simulink model "Fpump"  (R2025b)
settings: Solver=ode1be  StartTime=0.0  StopTime=300  FixedStep=0.03  RelTol=1e-3
undefined symbols (not defined in the file or in its folder): DiscIntNeverNeededParam
settings Model: Creator=peace  LastModifiedBy=peace
settings RTWCC: GPUComputeCapability=3.5

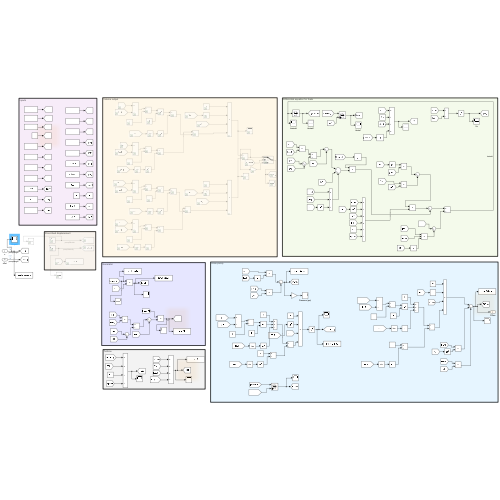
[thumbnail: Simulink's stored preview of the top-level diagram]
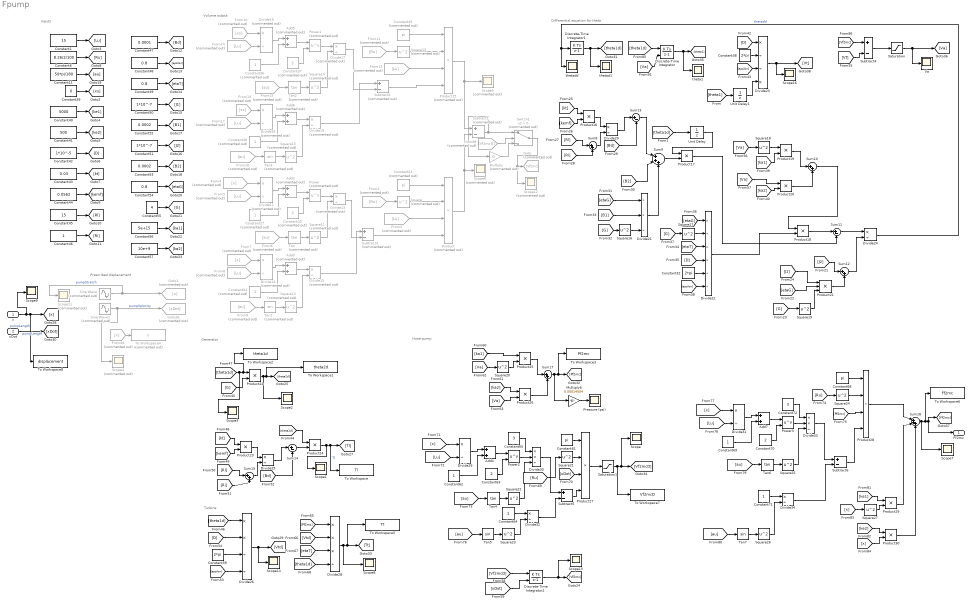
== system Fpump ==
  note: Turbine
  note: Hose-pump
  note: Generator
  note: Differential equation for theta
  note: Volume output
  note: Prescribed displacement
  note: Inputs
  x : Inport
  xDot : Inport  Port=2
  Add{2..3,5..6} (4 alike) : Sum  Commented=on
  Add4 : Sum
  Add7 : Sum
  Constant1 : Constant  Value=15
  Constant11 : Constant  Value=50*pi/180
  Constant23 : Constant  Commented=on  Value=pi
  Constant{27,34,36,38} (4 alike) : Constant  Commented=on
  Constant32 : Constant  Value=2*pi
  Constant33 : Constant  Commented=on  Value=3
  Constant35 : Constant  Commented=on  Value=pi
  Constant37 : Constant  Commented=on  Value=3
  Constant39 : Constant  Value=0
  Constant40 : Constant  Value=5000
  Constant41 : Constant  Value=500
  Constant42 : Constant  Value=1*10^-5
  Constant43 : Constant  Value=0.03
  Constant44 : Constant  Value=0.0562
  Constant45 : Constant  Value=15
  Constant{46,62,64,69,71} (5 alike) : Constant
  Constant47 : Constant  Value=0.0001
  Constant48 : Constant  Value=0.8
  Constant49 : Constant  Value=0.8
  Constant50 : Constant  Value=1*10^-7
  Constant51 : Constant  Value=1*10^-7
  Constant52 : Constant  Value=0.0002
  Constant53 : Constant  Value=0.0002
  Constant54 : Constant  Value=0.8
  Constant55 : Constant  Value=4
  Constant56 : Constant  Value=5e+15
  Constant57 : Constant  Value=10e+9
  Constant58 : Constant  Value=2*pi
  Constant59 : Constant  Value=2*pi
  Constant6 : Constant  Value=8.26/2/100
  Constant61 : Constant  Value=pi
  Constant63 : Constant  Value=2
  Constant65 : Constant  Value=3
  Constant68 : Constant  Value=pi
  Constant70 : Constant  Value=2
  Constant72 : Constant  Value=3
  Discrete-Time Integrator : DiscreteIntegrator  ExternalReset=falling  SampleTime=-1  ICPrevOutput=DiscIntNeverNeededParam  ICPrevScaledInput=DiscIntNeverNeededParam
  Discrete-Time Integrator1 : DiscreteIntegrator  SampleTime=-1  ICPrevOutput=DiscIntNeverNeededParam  ICPrevScaledInput=DiscIntNeverNeededParam
  Discrete-Time Integrator2 : DiscreteIntegrator  ExternalReset=falling  SampleTime=-1  ICPrevOutput=DiscIntNeverNeededParam  ICPrevScaledInput=DiscIntNeverNeededParam
  Divide{11,13..19} (8 alike) : Product  Commented=on  Inputs=*/
  Divide{20,24..25,29,31..32,34} (7 alike) : Product  Inputs=*/
  Divide21 : Product  Inputs=**/
  Divide22 : Product  Inputs=*/**//
  Divide23 : Product  Inputs=*//*
  Divide26 : Product  Inputs=**//
  Divide28 : Product  Inputs=***/
  Divide30 : Product  Inputs=**/
  Divide33 : Product  Inputs=**/
  From10 : From  Commented=on  GotoTag=xs
  From11 : From  Commented=on  GotoTag=Ru
  From{3,5,8,12,14,17} (6 alike) : From  Commented=on  GotoTag=Lu
  From13 : From  Commented=on  GotoTag=xs
  From{6,9,15,18} (4 alike) : From  Commented=on  GotoTag=au
  From2 : From  Commented=on  GotoTag=Ru
  From4 : From  Commented=on  GotoTag=x
  From64 : From  Commented=on  GotoTag=x
  From7 : From  Commented=on  GotoTag=x
  From89 : From  Commented=on  GotoTag=Vf2mcD
  Goto : Goto  Commented=on  GotoTag=Vf2mc
  Goto1 : Goto  Commented=on  GotoTag=x
  Goto26 : Goto  Commented=on  GotoTag=xDot
  Multiply : Gain  Commented=on  Gain=0
  Multiply6 : Gain  Gain=0.00014504
  Power : Math  Commented=on  Operator=pow
  Power1 : Math  Commented=on  Operator=pow
  Power2 : Math  Operator=pow
  Power3 : Math  Operator=pow
  Pressure (psi) : Scope
      settings: ActiveDisplayYMinimum=-78.359380613030112  ActiveDisplayYMaximum=705.23442551727112  DataLoggingVariableName=ScopeData10
  Product : Product  Commented=on  Inputs=4
  Product15 : Product  Commented=on  Inputs=4
  Product{16..20,22..26,29..30} (12 alike) : Product
  Product21 : Product  Inputs=3
  Product27 : Product  Inputs=4
  Product28 : Product  Inputs=4
  Saturation : Saturate  UpperLimit=Inf  LowerLimit=0
  Saturation1 : Saturate  UpperLimit=Inf  LowerLimit=0
  Scope{,1..3,7..9,13..14,16} (10 alike) : Scope
      Scope settings: ActiveDisplayYMinimum=-0.0003969816965604729  ActiveDisplayYMaximum=0.0035728352690442573  DataLoggingVariableName=ScopeData9
      Scope1 settings: ActiveDisplayYMinimum=-1  ActiveDisplayYMaximum=1
      Scope13 settings: ActiveDisplayYMinimum=-1  ActiveDisplayYMaximum=1  DataLoggingVariableName=ScopeData15
      Scope14 settings: ActiveDisplayYMinimum=-4.3E-5  ActiveDisplayYMaximum=4E-5  DataLoggingVariableName=ScopeData4
      Scope16 settings: ActiveDisplayYMinimum=-1  ActiveDisplayYMaximum=1  DataLoggingVariableName=ScopeData16
      Scope2 settings: ActiveDisplayYMinimum=-807.31564  ActiveDisplayYMaximum=7200.0744  DataLoggingVariableName=ScopeData2
      Scope3 settings: ActiveDisplayYMinimum=-201.82891  ActiveDisplayYMaximum=1800.0186  DataLoggingVariableName=ScopeData3
      Scope7 settings: ActiveDisplayYMinimum=-3.4318250735998834E+23  ActiveDisplayYMaximum=1.6249217794143435E+24  DataLoggingVariableName=ScopeData13
      Scope8 settings: ActiveDisplayYMinimum=-0.85985  ActiveDisplayYMaximum=7.73866  DataLoggingVariableName=ScopeData11
      Scope9 settings: DataLoggingVariableName=ScopeData7
  Scope{4..6,11..12} (5 alike) : Scope  Commented=on
      Scope11 settings: ActiveDisplayYMinimum=-0.24999999999999994  ActiveDisplayYMaximum=2.25  DataLoggingVariableName=ScopeData6
      Scope12 settings: ActiveDisplayYMinimum=-0.00094087179819930442  ActiveDisplayYMaximum=0.0084678461837937417  DataLoggingVariableName=ScopeData2
      Scope4 settings: ActiveDisplayYMinimum=-1  ActiveDisplayYMaximum=1
      Scope5 settings: ActiveDisplayYMinimum=0.07038  ActiveDisplayYMaximum=0.09038  DataLoggingVariableName=ScopeData5
      Scope6 settings: ActiveDisplayYMinimum=0.07191  ActiveDisplayYMaximum=0.08132  DataLoggingVariableName=ScopeData6
  Sine Wave : Sin  Commented=on  Bias=1  Frequency=2*pi/8  Phase=3*pi/2  SampleTime=0
  Sine Wave1 : Sin  Commented=on  Amplitude=1*2*pi/8  Frequency=2*pi/8  SampleTime=0
  Square{,11..15} (6 alike) : Math  Commented=on  Operator=square
  Square{16..27} (12 alike) : Math  Operator=square
  Subtract1 : Sum  Commented=on  Inputs=+-
  Subtract2 : Sum  Commented=on  Inputs=+-
  Subtract3 : Sum  Commented=on  Inputs=+-
  Subtract4 : Sum  Inputs=+-
  Subtract5 : Sum  Inputs=+-
  Subtract6 : Sum  Inputs=+-
  Sum{8,10,12,15,17} (5 alike) : Sum  Inputs=|++
  Sum11 : Sum  Inputs=|+-
  Sum13 : Sum  Inputs=|+-
  Sum14 : Sum  Inputs=|+-
  Sum18 : Sum  Inputs=|+++
  Sum9 : Sum  Inputs=|+++
  Switch1 : Switch  Commented=on  Criteria=u2 > Threshold  SaturateOnIntegerOverflow=off  InputSameDT=off
  Tan : Trigonometry  Commented=on  Operator=tan
  Tan1 : Trigonometry  Commented=on
  Tan2 : Trigonometry  Commented=on  Operator=tan
  Tan3 : Trigonometry  Commented=on
  Tan4 : Trigonometry  Operator=tan
  Tan5 : Trigonometry
  Tan6 : Trigonometry  Operator=tan
  Tan7 : Trigonometry
  To Workspace : ToWorkspace  VariableName=Tl  SampleTime=-1
  To Workspace1 : ToWorkspace  VariableName=theta2d  SampleTime=-1
  To Workspace2 : ToWorkspace  VariableName=theta1d  SampleTime=-1
  To Workspace3 : ToWorkspace  VariableName=Pf2mc  SampleTime=-1
  To Workspace4 : ToWorkspace  Commented=on  VariableName=x  SaveFormat=Structure With Time  SampleTime=-1
  To Workspace5 : ToWorkspace  VariableName=Tt  SampleTime=-1
  To Workspace6 : ToWorkspace  VariableName=Ff2mc  SampleTime=-1
  To Workspace7 : ToWorkspace  VariableName=Vf2mcD  SampleTime=-1
  To Workspace8 : ToWorkspace  VariableName=displacement  SampleTime=-1
  Unit Delay : UnitDelay  SampleTime=-1  HasFrameUpgradeWarning=on
  Unit Delay1 : UnitDelay  SampleTime=-1  HasFrameUpgradeWarning=on
  Va : Scope
      settings: ActiveDisplayYMinimum=-4E-6  ActiveDisplayYMaximum=3.2E-5  DataLoggingVariableName=ScopeData3
  theta1 : Scope
      settings: ActiveDisplayYMinimum=-472.7300411952894  ActiveDisplayYMaximum=4254.5703707576058  DataLoggingVariableName=ScopeData14
  thetad1 : Scope
      settings: ActiveDisplayYMinimum=-90.070687849635348  ActiveDisplayYMaximum=697.42712539466106  DataLoggingVariableName=ScopeData12
  thetadd : Scope
      settings: ActiveDisplayYMinimum=-1  ActiveDisplayYMaximum=1
  Ff2mc : Outport
  wires:
  Sine Wave/1 -> Scope11/1, Goto1/1  "pumpStretch"
  Constant11/1 -> [au]
  Constant1/1 -> [Lu]
  Constant6/1 -> [Ru]
  From2/1 -> Square/1
  Constant23/1 -> Product/1
  Square/1 -> Product/2
  From3/1 -> Product/3
  From5/1 -> Divide11/2
  Divide11/1 -> Add2/1
  Constant27/1 -> Add2/2
  Add2/1 -> Power/1
  Constant33/1 -> Power/2
  Power/1 -> Divide13/1
  From6/1 -> Tan/1
  Tan/1 -> Square11/1
  Square11/1 -> Divide13/2
  Tan1/1 -> Square12/1
  From9/1 -> Tan1/1
  Constant34/1 -> Add3/2
  Square12/1 -> Divide15/2
  From8/1 -> Divide14/2
  From7/1 -> Divide14/1
  Add3/1 -> Divide15/1
  Divide14/1 -> Add3/1
  Divide13/1 -> Subtract3/2
  Divide15/1 -> Subtract3/1
  Subtract3/1 -> Product/4
  Tan2/1 -> Square14/1
  Subtract2/1 -> Product15/4
  From15/1 -> Tan2/1
  From10/1 -> Divide16/1
  Divide19/1 -> Subtract2/1
  From14/1 -> Divide16/2
  Divide18/1 -> Add6/1
  From13/1 -> Divide18/1
  From17/1 -> Divide18/2
  Tan3/1 -> Square15/1
  Constant38/1 -> Add6/2
  From18/1 -> Tan3/1
  Constant37/1 -> Power1/2
  Square13/1 -> Product15/2
  Constant36/1 -> Add5/2
  Constant35/1 -> Product15/1
  From11/1 -> Square13/1
  Square14/1 -> Divide17/2
  Power1/1 -> Divide17/1
  Add5/1 -> Power1/1
  Add6/1 -> Divide19/1
  Square15/1 -> Divide19/2
  From12/1 -> Product15/3
  Divide16/1 -> Add5/1
  Product15/1 -> Subtract1/1, Scope5/1
  Constant39/1 -> [xs]
  From4/1 -> Divide11/1
  Divide17/1 -> Subtract2/2
  Product/1 -> Subtract1/2, Scope6/1
  Constant40/1 -> [ke1]
  Constant41/1 -> [ke2]
  Constant42/1 -> [D]
  Constant43/1 -> [kt]
  Constant44/1 -> [kemf]
  Constant46/1 -> [Ri]
  Constant47/1 -> [Bd]
  Constant45/1 -> [Rl]
  Constant48/1 -> [epsilon]
  Constant49/1 -> [etaT]
  Constant50/1 -> [J1]
  Constant52/1 -> [B1]
  Constant51/1 -> [J2]
  Constant53/1 -> [B2]
  Constant54/1 -> [etaG]
  Constant55/1 -> [G]
  [Rl] -> Sum8/1
  [Ri] -> Sum8/2
  [kt] -> Product16/1
  [kemf] -> Product16/2
  Product16/1 -> Divide20/1
  Sum8/1 -> Divide20/2
  Divide20/1 -> Sum13/1
  [Bd] -> Sum13/2
  [B2] -> Sum9/2
  [etaG] -> Divide21/1
  [G] -> Square16/1
  Square16/1 -> Divide21/3
  [B1] -> Divide21/2
  Sum9/1 -> Product17/2
  Square17/1 -> Divide22/2
  [G] -> Square17/1
  [etaG] -> Divide22/1
  [etaT] -> Divide22/3
  [D] -> Divide22/4
  Constant32/1 -> Divide22/5
  [epsilon] -> Divide22/6
  Constant56/1 -> [ka1]
  Constant57/1 -> [ka2]
  Divide22/1 -> Product18/2
  [D] -> Divide23/1
  [epsilon] -> Divide23/3
  Constant58/1 -> Divide23/2
  Square18/1 -> Product19/1
  [ka1] -> Product19/2
  [ka2] -> Product20/2
  Product19/1 -> Sum10/1
  Product20/1 -> Sum10/2
  Sum10/1 -> Product18/1
  Product18/1 -> Sum11/1
  Product17/1 -> Sum11/2
  Sum11/1 -> Divide24/1
  [J1] -> Product21/1
  [G] -> Square19/1
  [etaG] -> Product21/2
  Square19/1 -> Product21/3
  [J2] -> Sum12/1
  Product21/1 -> Sum12/2
  Sum12/1 -> Divide24/2
  Divide24/1 -> thetadd/1, Discrete-Time Integrator1/1  "thetadd"
  Subtract4/1 -> Saturation/1
  [theta1d] -> Scope3/1, To Workspace2/1, Product22/1
  [G] -> Product22/2
  Product22/1 -> Scope2/1, To Workspace1/1, [theta2d]
  Sum13/1 -> Sum9/1
  Divide21/1 -> Sum9/3
  [Ri] -> Sum15/2
  Product23/1 -> Divide25/1
  [Rl] -> Sum15/1
  [Bd] -> Sum14/2
  [kemf] -> Product23/2
  [kt] -> Product23/1
  Divide25/1 -> Sum14/1
  Sum15/1 -> Divide25/2
  Sum14/1 -> Product24/2
  Product24/1 -> Scope1/1, To Workspace/1, [Tl]  "Tl"
  [theta2d] -> Product24/1
  [theta1d] -> Divide26/1
  [D] -> Divide26/2
  Constant59/1 -> Divide26/3
  [epsilon] -> Divide26/4
  Divide26/1 -> Scope14/1, [Vtd]
  [Va] -> Square20/1
  [ka1] -> Product25/1
  Square20/1 -> Product25/2
  Product25/1 -> Sum17/1
  [ka2] -> Product26/1
  [Va] -> Product26/2
  Product26/1 -> Sum17/2
  Sum17/1 -> Multiply6/1, To Workspace3/1, [Pf2mc]
  From64/1 -> To Workspace4/1
  [Pf2mc] -> Divide28/1
  [Vtd] -> Divide28/2
  [etaT] -> Divide28/3
  [theta1d] -> Divide28/4
  Divide28/1 -> Scope8/1, To Workspace5/1, [Tt]
  Tan4/1 -> Square22/1
  Divide32/1 -> Subtract5/2
  [au] -> Tan4/1
  [Lu] -> Divide29/2
  Tan5/1 -> Square23/1
  Square21/1 -> Product27/2
  Constant62/1 -> Add4/2
  Constant64/1 -> Divide32/1
  Divide30/1 -> Subtract5/1
  [au] -> Tan5/1
  Square22/1 -> Divide30/3
  Constant61/1 -> Product27/1
  [Ru] -> Square21/1
  Power2/1 -> Divide30/2
  Add4/1 -> Power2/1
  [xDot] -> Product27/3
  [x] -> Divide29/1
  Constant63/1 -> Power2/2
  Divide29/1 -> Add4/1
  Constant65/1 -> Divide30/1
  Product27/1 -> Saturation1/1
  Saturation1/1 -> To Workspace7/1, Scope/1, [Vf2mcD]
  Multiply6/1 -> Pressure (psi)/1
  [Ru] -> Square24/1
  Constant72/1 -> Divide33/1
  [x] -> Divide31/1
  Add7/1 -> Power3/1
  [au] -> Tan7/1
  Divide31/1 -> Add7/1
  Constant70/1 -> Power3/2
  Constant71/1 -> Divide34/1
  Power3/1 -> Divide33/2
  Square26/1 -> Divide34/2
  [au] -> Tan6/1
  Square25/1 -> Divide33/3
  [Lu] -> Divide31/2
  Divide34/1 -> Subtract6/2
  Tan6/1 -> Square25/1
  Constant69/1 -> Add7/2
  Tan7/1 -> Square26/1
  Divide33/1 -> Subtract6/1
  Constant68/1 -> Product28/1
  Square24/1 -> Product28/2
  [Pf2mc] -> Product28/3
  Subtract6/1 -> Product28/4
  [ke1] -> Product29/1
  [x] -> Square27/1
  Square27/1 -> Product29/2
  [ke2] -> Product30/1
  [x] -> Product30/2
  Product28/1 -> Sum18/1
  Product29/1 -> Sum18/2
  Product30/1 -> Sum18/3
  Subtract5/1 -> Product27/4
  Square23/1 -> Divide32/2
  [theta1] -> Unit Delay1/1
  [theta1d] -> Unit Delay/1
  Sine Wave1/1 -> Scope4/1, Goto26/1  "pumpVelocity"
  [Va] -> Square18/1
  [Va] -> Product20/1
  Saturation/1 -> [Va], Va/1
  [Vt] -> Subtract4/2
  Discrete-Time Integrator1/1 -> thetad1/1, [theta1d]
  [theta1d] -> Discrete-Time Integrator/1
  Discrete-Time Integrator/1 -> [theta1], theta1/1
  [Vf2mc] -> Subtract4/1
  Divide23/1 -> [Vt], Scope16/1
  Subtract1/1 -> Multiply/1, Switch1/1
  Switch1/1 -> Scope12/1, Goto/1
  From89/1 -> Switch1/2
  Multiply/1 -> Switch1/3
  [Va] -> Discrete-Time Integrator/2
  [Vf2mcD] -> Discrete-Time Integrator2/1
  Discrete-Time Integrator2/1 -> [Vf2mc], Scope13/1
  [xDot] -> Discrete-Time Integrator2/2
  Sum18/1 -> Scope7/1, To Workspace6/1, [Ff2mc], Ff2mc/1
  x/1 -> Scope9/1, To Workspace8/1, [x]  "pumpLength"
  xDot/1 -> [xDot]  "pumpLength"
  Unit Delay/1 -> Product17/1
  Unit Delay1/1 -> Divide23/4
